simulink model "Signal_Modulation"  (R2020a)
settings: Solver=ode45  StartTime=0.0  StopTime=0.1  MaxStep=1e-6
libraries: commanapbnd3 x2, dsparch4 x1
settings Model: Creator=Gleb  LastModifiedBy=Gleb

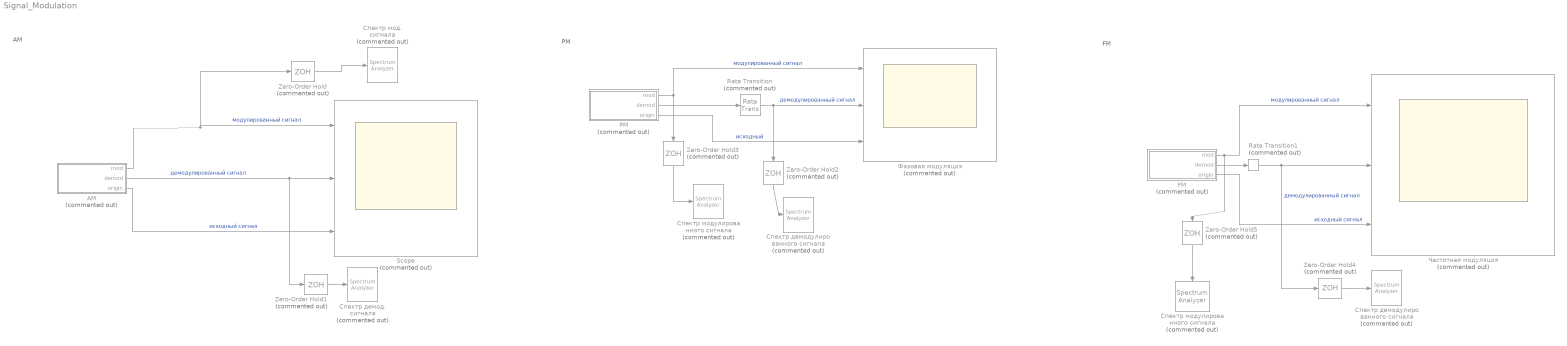
== system Signal_Modulation ==
  note: FM
  note: PM
  note: AM
  AM : Subsystem  Commented=on  mask{m=0.5, Uc=1000, Um=100}
      mask prompts: m "коэффициент модуляции"; Uc "частота несущей,Гц"; Um "частота мод.,Гц"
  FM : Subsystem  Commented=on  mask{Uc=1000, Um=100, wd=500}
      mask prompts: Uc "несущая частота, Гц"; Um "модул. частота, Гц"; wd "девиация частоты, Гц"
  PM : Subsystem  Commented=on  mask{Uc=1000, Um=100, m=2}
      mask prompts: Uc "несущая частота, Гц"; Um "модул. частота, Гц"; m "коэффициент модуляции"
  Rate Transition : RateTransition  Commented=on
  Rate Transition1 : RateTransition  Commented=on
  Scope : Scope  Commented=on  NumInputPorts=3
  Zero-Order Hold{,1..5} (6 alike) : ZeroOrderHold  Commented=on  SampleTime=-1
  Спектр демод. сигнала : SpectrumAnalyzer  Commented=on
  Спектр демодулированного сигнала : SpectrumAnalyzer  Commented=on
  "Спектр демодулированного сигнала " : SpectrumAnalyzer  Commented=on
  Спектр мод. сигнала : SpectrumAnalyzer  Commented=on
  Спектр модулированного сигнала : SpectrumAnalyzer  Commented=on
  "Спектр модулированного сигнала " : SpectrumAnalyzer  Commented=on
  Фазовая модуляция : Scope  Commented=on  NumInputPorts=3
  Частотная модуляция : Scope  Commented=on  NumInputPorts=3
  wires:
  AM/1(mod) -> Zero-Order Hold/1, Scope/1  "модулированный сигнал"
  AM/2(demod) -> Zero-Order Hold1/1, Scope/2  "демодулированный сигнал"
  AM/3(origin) -> Scope/3  "исходный сигнал"
  PM/1(mod) -> Zero-Order Hold3/1, Фазовая модуляция/1  "модулированный сигнал"
  Zero-Order Hold/1 -> Спектр мод. сигнала/1
  Zero-Order Hold1/1 -> Спектр демод. сигнала/1
  PM/3(origin) -> Фазовая модуляция/3  "исходный"
  PM/2(demod) -> Rate Transition/1
  Rate Transition/1 -> Фазовая модуляция/2, Zero-Order Hold2/1  "демодулированный сигнал"
  Zero-Order Hold2/1 -> "Спектр демодулированного сигнала "/1
  FM/3(origin) -> Частотная модуляция/3  "исходный сигнал"
  FM/2(demod) -> Rate Transition1/1
  FM/1(mod) -> Zero-Order Hold5/1, Частотная модуляция/1  "модулированный сигнал"
  Rate Transition1/1 -> Zero-Order Hold4/1, Частотная модуляция/2  "демодулированный сигнал"
  Zero-Order Hold3/1 -> "Спектр модулированного сигнала "/1
  Zero-Order Hold4/1 -> Спектр демодулированного сигнала/1
  Zero-Order Hold5/1 -> Спектр модулированного сигнала/1

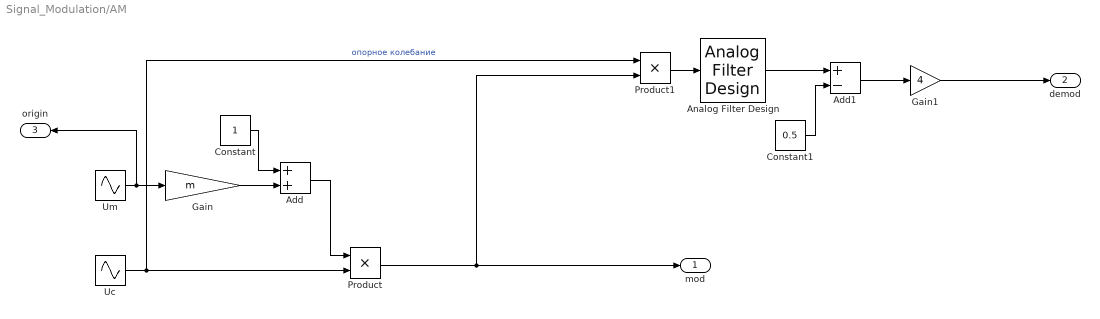
== system Signal_Modulation/AM ==
  Add : Sum
  Add1 : Sum  Inputs=+-
  Analog Filter Design : dsparch4/Analog Filter Design  method=Butterworth  filttype=Lowpass  N=8  Wlo=6283.200  Whi=80  Rp=2  Rs=40
  Constant : Constant
  Constant1 : Constant  Value=0.5
  Gain : Gain  Gain=m
  Gain1 : Gain  Gain=4
  Product : Product
  Product1 : Product
  Uc : Sin  Frequency=2*pi*Uc  Phase=pi/2  SampleTime=0
  Um : Sin  Frequency=2*pi*Um  Phase=pi/2  SampleTime=0
  mod : Outport
  demod : Outport  Port=2
  origin : Outport  Port=3
  wires:
  Uc/1 -> Product1/1, Product/2  "опорное колебание"
  Um/1 -> origin/1, Gain/1
  Gain/1 -> Add/2
  Constant/1 -> Add/1
  Add/1 -> Product/1
  Product/1 -> Product1/2, mod/1
  Product1/1 -> Analog Filter Design/1
  Constant1/1 -> Add1/2
  Analog Filter Design/1 -> Add1/1
  Add1/1 -> Gain1/1
  Gain1/1 -> demod/1

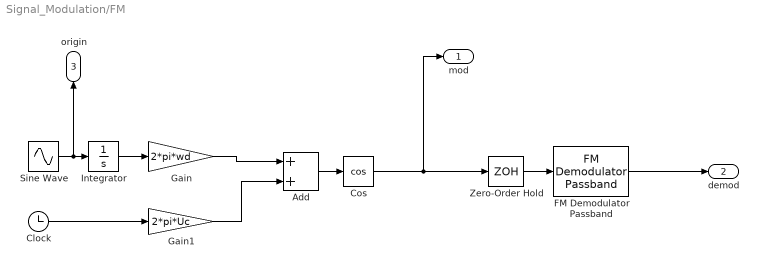
== system Signal_Modulation/FM ==
  Add : Sum
  Clock : Clock
  Cos : Trigonometry  Operator=cos
  FM Demodulator Passband : commanapbnd3/FM Demodulator Passband  Fc=Uc  Ph=0  Kc=wd  Ho=100
      settings: SourceProductBaseCode=CM
  Gain : Gain  Gain=2*pi*wd
  Gain1 : Gain  Gain=2*pi*Uc
  Integrator : Integrator
  Sine Wave : Sin  Frequency=2*pi*Um  Phase=pi/2  SampleTime=0
  Zero-Order Hold : ZeroOrderHold  SampleTime=1e-4
  mod : Outport
  demod : Outport  Port=2
  origin : Outport  Port=3
  wires:
  Gain1/1 -> Add/2
  Gain/1 -> Add/1
  Add/1 -> Cos/1
  Cos/1 -> mod/1, Zero-Order Hold/1
  Clock/1 -> Gain1/1
  Sine Wave/1 -> origin/1, Integrator/1
  Integrator/1 -> Gain/1
  Zero-Order Hold/1 -> FM Demodulator Passband/1
  FM Demodulator Passband/1 -> demod/1

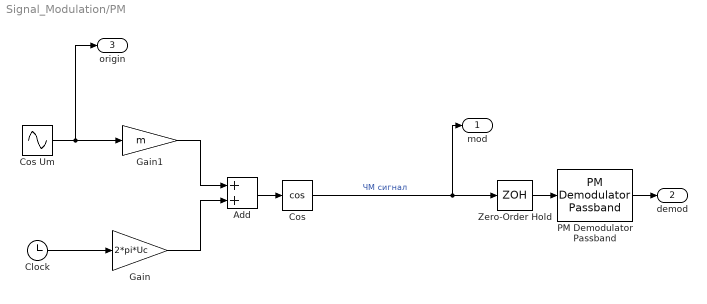
== system Signal_Modulation/PM ==
  Add : Sum
  Clock : Clock
  Cos : Trigonometry  Operator=cos
  Cos Um : Sin  Frequency=2*pi*Um  Phase=pi/2  SampleTime=0
  Gain : Gain  Gain=2*pi*Uc
  Gain1 : Gain  Gain=m
  PM Demodulator Passband : commanapbnd3/PM Demodulator Passband  Fc=1000  Ph=0  Kc=m  Ho=100
      settings: SourceProductBaseCode=CM
  Zero-Order Hold : ZeroOrderHold  SampleTime=1e-4
  mod : Outport
  demod : Outport  Port=2
  origin : Outport  Port=3
  wires:
  Cos Um/1 -> Gain1/1, origin/1
  Cos/1 -> mod/1, Zero-Order Hold/1  "ЧМ сигнал"
  Zero-Order Hold/1 -> PM Demodulator Passband/1
  PM Demodulator Passband/1 -> demod/1
  Clock/1 -> Gain/1
  Gain/1 -> Add/2
  Gain1/1 -> Add/1
  Add/1 -> Cos/1
